simulink model "final_project"  (R2021b)
settings: Solver=ode3  StartTime=0.0  StopTime=400  FixedStep=0.5  RelTol=1e-3  EnableMultiTasking=on
undefined symbols (not defined in the file): DiscIntNeverNeededParam
libraries: arduinolib x3, simulink x1
settings Model: ExtModeTrigDuration=2  Creator=madip  LastModifiedBy=arvt
settings DataIOCC: SaveOutput=off  SignalLogging=off  DSMLogging=off  SaveTime=off  ReturnWorkspaceOutputs=off
settings OptimizationCC: StrengthReduction=on  PassReuseOutputArgsAs=Individual arguments  ZeroExternalMemoryAtStartup=off  ZeroInternalMemoryAtStartup=off  MaxStackSize=64  OptimizeBlockOrder=speed  OptimizationPriority=Speed  OptimizationCustomize=off  MultiThreadedLoops=on  EfficientTunableParamExpr=on
settings DebuggingCC: ParameterTunabilityLossMsg=error
settings HardwareCC: ProdBitPerInt=16  ProdBitPerPointer=16  ProdBitPerSizeT=16  ProdBitPerPtrDiffT=16  ProdLargestAtomicFloat=None  ProdWordSize=8  ProdHWDeviceType=Atmel->AVR
settings SFSimCC: MATLABDynamicMemAlloc=off
settings RTWCC: Description=Embedded Coder  SystemTargetFile=ert.tlc  HardwareBoard=Arduino Leonardo  TemplateMakefile=ert_default_tmf  Toolchain=Arduino AVR  BuildConfiguration=Faster Runs
settings CodeAppCC: ForceParamTrailComments=on  IgnoreCustomStorageClasses=off  OperatorAnnotations=on  SimulinkDataObjDesc=on  SFDataObjDesc=on  InsertBlockDesc=on
settings ERTTargetCC: SupportContinuousTime=on  SupportVariableSizeSignals=on  ExtModeTransport=5  ExtModeStaticAllocSize=250  ExtModeMexFile=ext_serial_win32_comm_leonardo

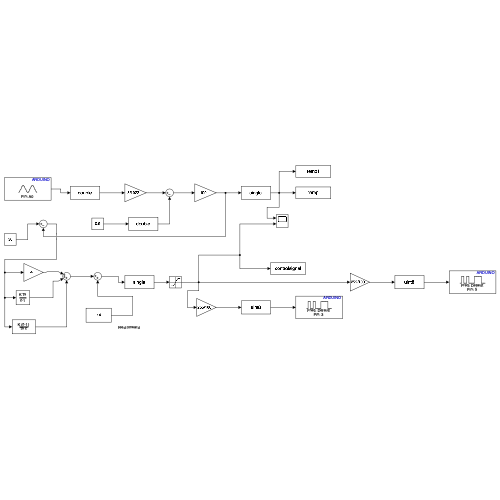
[thumbnail: Simulink's stored preview of the top-level diagram]
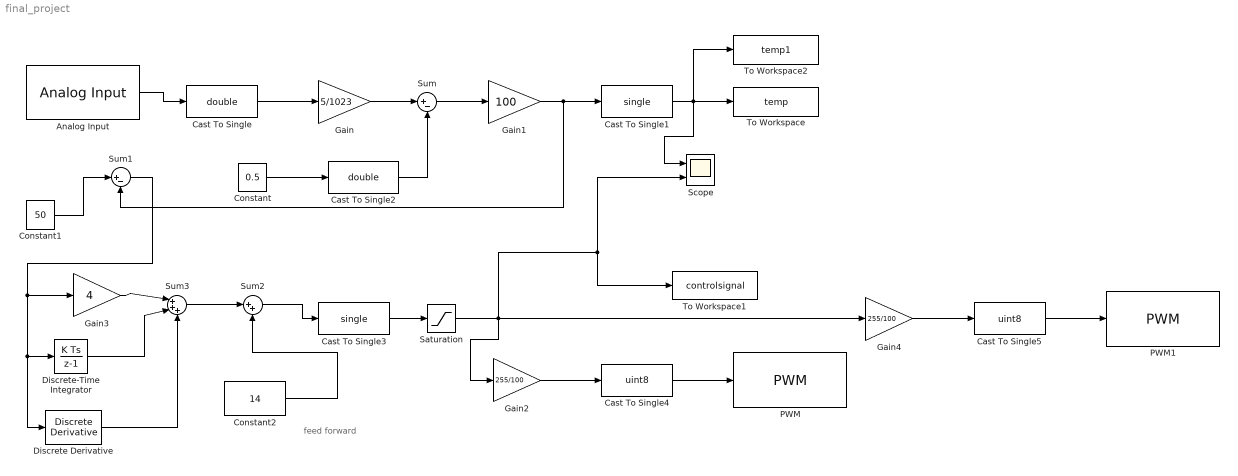
== system final_project ==
  note: feed forward
  Analog Input : arduinolib/Analog Input  pinNumber=0  ReadResultsOnly=off  ConversionTriggerSource=Software  ExternalTriggerType=uint32( 0 )  OutputDataType=uint16  EnableConversionCompleteNotify=off  EnableOuputStatus=off  SampleTime=0.5  blockPlatform=arduino
  Cast To Single : DataTypeConversion  OutDataTypeStr=double
  Cast To Single1 : DataTypeConversion  OutDataTypeStr=single
  Cast To Single2 : DataTypeConversion  OutDataTypeStr=double
  Cast To Single3 : DataTypeConversion  OutDataTypeStr=single
  Cast To Single4 : DataTypeConversion  OutDataTypeStr=uint8
  Cast To Single5 : DataTypeConversion  OutDataTypeStr=uint8
  Constant : Constant  Value=0.5  SampleTime=0.5
  Constant1 : Constant  Value=50  SampleTime=0.5
  Constant2 : Constant  Value=14  SampleTime=0.5
  Discrete Derivative : simulink/Discrete/Discrete Derivative  gainval=2  ICPrevScaledInput=0.0  OutMin=[]  OutMax=[]  OutDataType=fixdt(1, 16)  OutScaling=2^-10  DoSatur=off
  Discrete-Time Integrator : DiscreteIntegrator  gainval=0.1  SampleTime=0.5  ICPrevOutput=DiscIntNeverNeededParam  ICPrevScaledInput=DiscIntNeverNeededParam
  Gain : Gain  Gain=5/1023
  Gain1 : Gain  Gain=100
  Gain2 : Gain  Gain=255/100
  Gain3 : Gain  Gain=4
  Gain4 : Gain  Gain=255/100
  PWM : arduinolib/PWM  pinNumber=3  frequencyType=Default  desiredFrequency=490.2  achievableFrequency=490.2
  PWM1 : arduinolib/PWM  pinNumber=5  frequencyType=Default  desiredFrequency=490.2  achievableFrequency=490.2
  Saturation : Saturate  UpperLimit=100  LowerLimit=0
  Scope : Scope  NumInputPorts=2
  Sum : Sum  Inputs=|+-
  Sum1 : Sum  Inputs=|+-
  Sum2 : Sum  Inputs=|++
  Sum3 : Sum  Inputs=|+++
  To Workspace : ToWorkspace  VariableName=temp  SampleTime=0.5
      settings: Save2DSignal=2-D array (concatenate along first dimension)
  To Workspace1 : ToWorkspace  VariableName=controlsignal  SampleTime=0.5
      settings: Save2DSignal=2-D array (concatenate along first dimension)
  To Workspace2 : ToWorkspace  VariableName=temp1  SampleTime=0.5
      settings: Save2DSignal=2-D array (concatenate along first dimension)
  wires:
  Analog Input/1 -> Cast To Single/1
  Cast To Single/1 -> Gain/1
  Gain/1 -> Sum/1
  Sum/1 -> Gain1/1
  Gain1/1 -> Cast To Single1/1, Sum1/2
  Cast To Single2/1 -> Sum/2
  Constant/1 -> Cast To Single2/1
  Constant1/1 -> Sum1/1
  Cast To Single1/1 -> To Workspace2/1, Scope/1, To Workspace/1
  Cast To Single3/1 -> Saturation/1
  Gain2/1 -> Cast To Single4/1
  Cast To Single4/1 -> PWM/1
  Sum2/1 -> Cast To Single3/1
  Constant2/1 -> Sum2/2
  Sum3/1 -> Sum2/1
  Gain3/1 -> Sum3/1
  Sum1/1 -> Discrete Derivative/1, Discrete-Time Integrator/1, Gain3/1
  Discrete-Time Integrator/1 -> Sum3/2
  Discrete Derivative/1 -> Sum3/3
  Gain4/1 -> Cast To Single5/1
  Cast To Single5/1 -> PWM1/1
  Saturation/1 -> Gain4/1, Scope/2, To Workspace1/1, Gain2/1
